simulink model "fig9_86"  (Simulink 4.00)
settings: Solver=ode45  SolverMode=SingleTasking  StartTime=0.0  StopTime=100.0  RelTol=1e-3  AbsTol=1e-6
values from neighbouring files (symbols this model uses):
  a = 1    [fig3_18.m]    (also in fig3_31.m; fig3_32a.m; fig3_32b.m = 0.5; fig3_32c.m = 0.5)
undefined symbols (not defined in the file or in its folder): b, c, d, k1, ko, ll
libraries: simulink3 x1
CloseFcn:
  | ;slview('closediagram',bdroot);
settings Model: LastModifiedBy=abbas  LimitDataPoints=off  ExtModeTrigMode=oneshot  ExtModeArmWhenConnect=off  BlockReductionOpt=off

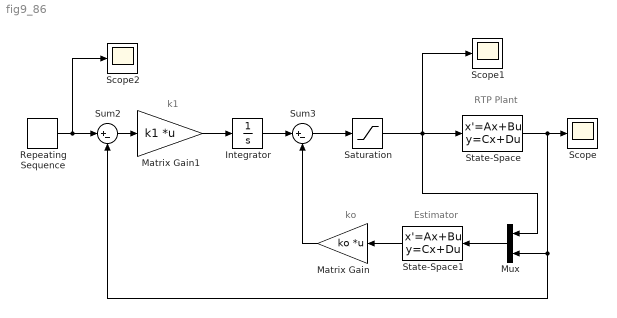
== system fig9_86 ==
  note: ko
  note: k1
  note: Estimator
  note: RTP Plant
  Integrator : Integrator  ExternalReset=none  InitialConditionSource=internal  InitialCondition=0  LimitOutput=off  UpperSaturationLimit=inf  LowerSaturationLimit=-inf  ShowSaturationPort=off  ShowStatePort=off  AbsoluteTolerance=auto
  Matrix Gain : Gain  Orientation=left  Gain=ko  Multiplication=Matrix(K*u)  SaturateOnIntegerOverflow=on
  Matrix Gain1 : Gain  Gain=k1  Multiplication=Matrix(K*u)  SaturateOnIntegerOverflow=on
  Mux : Mux  Orientation=left  Inputs=2
  Repeating Sequence : simulink3/Sources/Repeating Sequence  rep_seq_t=[0:0.1:100]  rep_seq_y=[0:.1:25 25*ones(1,500) 0*ones(1,250)]
  Saturation : Saturate  UpperLimit=10  LowerLimit=0  LinearizeAsGain=on
  Scope : Scope
      settings: TickLabels=on  TimeRange=auto  YMin=-5  YMax=5  SaveToWorkspace=off  SaveName=ScopeData  DataFormat=Array  LimitDataPoints=on  MaxDataPoints=5000
  Scope1 : Scope
      settings: TickLabels=on  TimeRange=auto  YMin=-5  YMax=5  SaveToWorkspace=off  SaveName=ScopeData  DataFormat=Array  LimitDataPoints=on  MaxDataPoints=5000
  Scope2 : Scope
      settings: TickLabels=on  TimeRange=auto  YMin=-5  YMax=5  SaveToWorkspace=off  SaveName=ScopeData  DataFormat=Array  LimitDataPoints=on  MaxDataPoints=5000
  State-Space : StateSpace  A=a  B=b  C=c  D=d  X0=0  Realization=auto  AbsoluteTolerance=auto
  State-Space1 : StateSpace  Orientation=left  A=a-ll*c  B=[b ll]  C=eye(3)  D=0*ones(3,2)  X0=0  Realization=auto  AbsoluteTolerance=auto
  Sum2 : Sum  Inputs=|+-  SaturateOnIntegerOverflow=on
  Sum3 : Sum  Inputs=|+-  SaturateOnIntegerOverflow=on
  wires:
  Matrix Gain1/1 -> Integrator/1
  Integrator/1 -> Sum3/1
  Sum3/1 -> Saturation/1
  Saturation/1 -> State-Space/1, Scope1/1, Mux/1
  Repeating Sequence/1 -> Scope2/1, Sum2/1
  State-Space/1 -> Scope/1, Mux/2, Sum2/2
  State-Space1/1 -> Matrix Gain/1
  Mux/1 -> State-Space1/1
  Matrix Gain/1 -> Sum3/2
  Sum2/1 -> Matrix Gain1/1
